simulink model "Synchronous_Buck_Converter_V2016B"  (R2016b)
settings: Solver=VariableStepAuto  StartTime=0.0  StopTime=0.006  RelTol=1e-3
libraries: fl_lib x13, elec_lib x7, nesl_utility x5
settings Model: Creator=whl14  LastModifiedBy=whl14

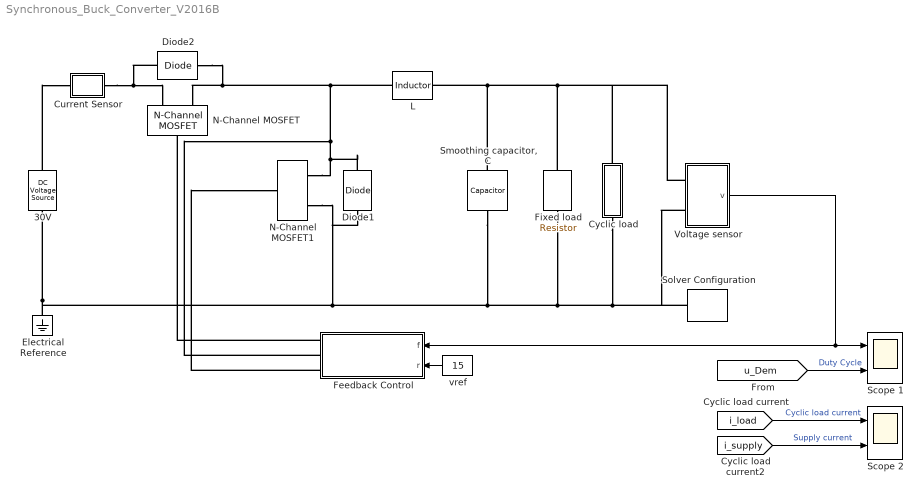
== system Synchronous_Buck_Converter_V2016B ==
  30V : fl_lib/Electrical/Electrical Sources/DC Voltage Source  v0=30 V
  Current Sensor : Subsystem
  Cyclic load : Subsystem
  Diode1 : elec_lib/Semiconductor Devices/Diode  ModelType=3  Vf=0.6 V  Ron=0.3 Ohm  Goff=1e-8 S  Rz=0.3 Ohm  Vz=50 V  C_PWL=5 pF  prmExp=1  I12=[ 0.25 5 ] A  V12=[ 0.7 0.8 ] V  I1=0.0137 A  V1=0.6 V  RS=0.01 Ohm  IS=1e-12 A  Tmeas=25 degC  ec=1  BV=Inf V  C_param=1  CJ0=5 pF  VJ=1 V  Mgrad=0.5  Vvec=[ 0.1 10 100 ] V  Cvec=[ 3.5 1 0.4 ] pF  FC=0.5  Q_param=1  Irrm=-7.15 A  iF=4 A  didt=-750 A/us  trr=115 ns  TT=50 ns  tau=100 ns  T_param=1  IS_T2=1.25e-7 A  I1_T2=0.245 A  V1_T2=0.5 V  Tmeas2=125 degC  EG_param=1  EG=1.11 eV  XTI_param=1  XTI=3  dBVdT=0 V/K  Tdevice=25 degC  Rth=[ 0 10 ] K/W  thermal_mass_parameterization=1  thermal_mass=[ 0 1 ] J/K  thermal_time_constant=[ 0 10 ] s  thermal_mass_initial_temperatures=[ 25 25 ] degC
  Diode2 : elec_lib/Semiconductor Devices/Diode  ModelType=3  Vf=0.6 V  Ron=0.3 Ohm  Goff=1e-8 S  Rz=0.3 Ohm  Vz=50 V  C_PWL=5 pF  prmExp=1  I12=[ 0.25 5 ] A  V12=[ 0.7 0.8 ] V  I1=0.0137 A  V1=0.6 V  RS=0.01 Ohm  IS=1e-12 A  Tmeas=25 degC  ec=1  BV=Inf V  C_param=1  CJ0=5 pF  VJ=1 V  Mgrad=0.5  Vvec=[ 0.1 10 100 ] V  Cvec=[ 3.5 1 0.4 ] pF  FC=0.5  Q_param=1  Irrm=-7.15 A  iF=4 A  didt=-750 A/us  trr=115 ns  TT=50 ns  tau=100 ns  T_param=1  IS_T2=1.25e-7 A  I1_T2=0.245 A  V1_T2=0.5 V  Tmeas2=125 degC  EG_param=1  EG=1.11 eV  XTI_param=1  XTI=3  dBVdT=0 V/K  Tdevice=25 degC  Rth=[ 0 10 ] K/W  thermal_mass_parameterization=1  thermal_mass=[ 0 1 ] J/K  thermal_time_constant=[ 0 10 ] s  thermal_mass_initial_temperatures=[ 25 25 ] degC
  Electrical Reference : fl_lib/Electrical/Electrical Elements/Electrical Reference
  Feedback Control : Subsystem  mask{Kp=0.5, Ki=200}
      mask init:
      | Kp=0.5
      | Ki=200
  Fixed load : fl_lib/Electrical/Electrical Elements/Resistor  R=3.75 Ohm  i_specify=off  i_priority=None  i=0 A  v_specify=off  v_priority=None  v=0 V
  L : fl_lib/Electrical/Electrical Elements/Inductor  l=1e-3 H  r=0 Ohm  g=0 1/Ohm  i_specify=off  i_priority=None  i=0 A  v_specify=off  v_priority=None  v=0 V  i_L_specify=off  i_L_priority=High  i_L=0 A
      settings: LogSimulationData=on
  N-Channel MOSFET : elec_lib/Semiconductor Devices/N-Channel MOSFET  parameterization=1  prmDatasheet=2  prmEquCoeff=1  Beta=5 A/V^2  Rds=0.1 Ohm  Id=6 A  Vgs=15 V  Vth=2 V  lam=0 1/V  Tmeas=25 degC  RS=0.01 Ohm  RD=0.01 Ohm  C_param=1  C_GS=270 pF  C_GD=80 pF  C_DS=0 pF  C_iss=350 pF  C_rss=80 pF  C_oss=0 pF  C_GS_vec=[ 270 300 290 280 295 255 ] pF  C_GD_vec=[ 450 400 300 190 95 55 ] pF  C_DS_vec=[ 450 410 390 230 175 115 ] pF  C_iss_vec=[ 720 700 590 470 390 310 ] pF  C_rss_vec=[ 450 400 300 190 95 55 ] pF  C_oss_vec=[ 900 810 690 420 270 170 ] pF  C_Vds_vec=[ 0.1 0.3 1 3 10 30 ] V  charge_linearity_param=1  C_OX=200 pF  V_C_OX=-0.5 V  IsDiode=0 A  Vbi=0.6 V  n=1  Cj0Diode=0 pF  TT=50e-9 s  dVth_dT=-6 mV/K  Rds_T2=0.2 Ohm  Tmeas2=125 degC  BEXDatasheet=-1.5  BEXEquCoeff=-1.5  etaisDatasheet=3  etaisEquCoeff=3  TdeviceDatasheet=T_junction1 degC  TdeviceEquCoeff=25 degC  Rth=[1.0, 10.0] K/W  thermal_mass_parameterization=1  thermal_mass=[1.0, 1.0] J/K  thermal_time_constant=[1.0, 10.0] s  thermal_mass_initial_temperatures=[ 25 25 ] degC  betaref=18 A/V^2  Vfbref=-1.1 V  gamma=3.5 V^0.50000  phib2ref=1 V  thesatref=0.4 1/V  alpha=0  Vp=5e-2 V  m=8  Tref=25 degC  Cox=1500 pF  Cgso=100 pF  Cgdo=14 pF  Rsref=2e-3 Ohm  Rdref=0.17 Ohm  Rgref=8.4 Ohm  Isref=5.2e-13 A  Cj0=480 pF  Tprm=1  etabet=1.3  Stvfb=5e-4 V/K  Stphib=-8.5e-4 V/K  etasat=1.04  etar=0.95  etais=3  Tsim=25 degC  T0=[25.0, 25.0] degC
  N-Channel MOSFET1 : elec_lib/Semiconductor Devices/N-Channel MOSFET  parameterization=1  prmDatasheet=1  prmEquCoeff=1  Beta=5 A/V^2  Rds=0.1 Ohm  Id=6 A  Vgs=15 V  Vth=2 V  lam=0 1/V  Tmeas=25 degC  RS=1e-4 Ohm  RD=0.01 Ohm  C_param=1  C_GS=270 pF  C_GD=80 pF  C_DS=0 pF  C_iss=350 pF  C_rss=80 pF  C_oss=0 pF  C_GS_vec=[ 270 300 290 280 295 255 ] pF  C_GD_vec=[ 450 400 300 190 95 55 ] pF  C_DS_vec=[ 450 410 390 230 175 115 ] pF  C_iss_vec=[ 720 700 590 470 390 310 ] pF  C_rss_vec=[ 450 400 300 190 95 55 ] pF  C_oss_vec=[ 900 810 690 420 270 170 ] pF  C_Vds_vec=[ 0.1 0.3 1 3 10 30 ] V  charge_linearity_param=1  C_OX=200 pF  V_C_OX=-0.5 V  IsDiode=0 A  Vbi=0.6 V  n=1  Cj0Diode=0 pF  TT=50e-9 s  dVth_dT=-6 mV/K  Rds_T2=0.037 Ohm  Tmeas2=125 degC  BEXDatasheet=-1.5  BEXEquCoeff=-1.5  etaisDatasheet=3  etaisEquCoeff=3  TdeviceDatasheet=25 degC  TdeviceEquCoeff=25 degC  Rth=[1.0, 10.0] K/W  thermal_mass_parameterization=1  thermal_mass=[1.0, 1.0] J/K  thermal_time_constant=[1.0, 10.0] s  thermal_mass_initial_temperatures=[ 25 25 ] degC  betaref=18 A/V^2  Vfbref=-1.1 V  gamma=3.5 V^0.50000  phib2ref=1 V  thesatref=0.4 1/V  alpha=0  Vp=5e-2 V  m=8  Tref=25 degC  Cox=1500 pF  Cgso=100 pF  Cgdo=14 pF  Rsref=2e-3 Ohm  Rdref=0.17 Ohm  Rgref=8.4 Ohm  Isref=5.2e-13 A  Cj0=480 pF  Tprm=1  etabet=1.3  Stvfb=5e-4 V/K  Stphib=-8.5e-4 V/K  etasat=1.04  etar=0.95  etais=3  Tsim=25 degC  T0=[25.0, 25.0] degC
  Scope 1 : Scope  NumInputPorts=2
  Scope 2 : Scope  NumInputPorts=2
  "Smoothing capacitor, C" : fl_lib/Electrical/Electrical Elements/Capacitor  c=22 uF  r=0 Ohm  g=0 1/Ohm  i_specify=off  i_priority=None  i=0 A  v_specify=off  v_priority=None  v=0 V  vc_specify=on  vc_priority=High  vc=0 V
  Solver Configuration : nesl_utility/Solver Configuration  PhysicalDomain=network_engine_domain  SubClassName=solver  LeftPortType=input  RightPortType=generic  Accelerate=off  Tones=[]  Harmonics=[]  SimulateNoise=off  Profile=off  UseLocalSampling=off  EnableSwitchedLinearOptims=on  FrequencyDomain=off  UseCCode=off  RelTol=0.001  AbsTol=1e-06  MinStep=1e-09  ToWorkspace=off  RevertToSquareIcSolve=off  NumHomotopyIterations=100  PhasorMode=off  PhasorModeNumHarmonics=1  OverrideAbsTol=off  DoDC=off  ResidualTolerance=1e-09  UseLocalSolver=off  LocalSolverChoice=NE_BACKWARD_EULER_ADVANCER  LocalSolverSampleTime=0.001  DoFixedCost=off  MaxNonlinIter=3  MaxModeIter=2  LinearAlgebra=Sparse  DelaysMemoryBudget=1024  AutomaticFiltering=on  FilteringTimeConstant=0.001
  Voltage sensor : Subsystem
  vref : Constant  Value=15
  wires:
  Voltage sensor/1(v) -> Feedback Control/1(f), Scope 1/1
  [i_load] -> Scope 2/1  "Cyclic load current"
  [i_supply] -> Scope 2/2  "Supply current"
  [u_Dem] -> Scope 1/2  "Duty Cycle"
  vref/1 -> Feedback Control/2(r)
  connections:
  Current Sensor/RConn1 -- Diode2/RConn1 -- N-Channel MOSFET/RConn1
  30V/LConn1 -- Current Sensor/LConn1
  N-Channel MOSFET1/RConn1 -- Diode1/RConn1 -- Feedback Control/RConn2 -- L/LConn1 -- Diode2/LConn1 -- N-Channel MOSFET/RConn2
  Electrical Reference/LConn1 -- "Smoothing capacitor, C"/RConn1 -- Fixed load/RConn1 -- Voltage sensor/LConn2 -- Solver Configuration/RConn1 -- Cyclic load/LConn1 -- Diode1/LConn1 -- N-Channel MOSFET1/RConn2 -- 30V/RConn1
  "Smoothing capacitor, C"/LConn1 -- Voltage sensor/LConn1 -- Cyclic load/RConn1 -- Fixed load/LConn1 -- L/RConn1
  Feedback Control/RConn1 -- N-Channel MOSFET/LConn1
  Feedback Control/RConn3 -- N-Channel MOSFET1/LConn1

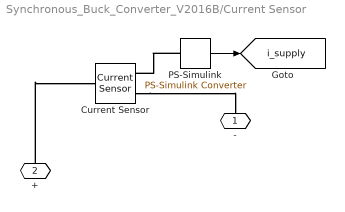
== system Synchronous_Buck_Converter_V2016B/Current Sensor ==
  Current Sensor : fl_lib/Electrical/Electrical Sensors/Current Sensor
  PS-Simulink : nesl_utility/PS-Simulink Converter  PhysicalDomain=network_engine_domain  SubClassName=ps_output  LeftPortType=input  RightPortType=output  PseudoPeriodic=off  Frequencies=[]  Unit=1  AffineConversion=off
  - : PMIOPort  Port=1  Side=Right
  + : PMIOPort  Port=2  Side=Left
  tag scope: i_supply=global
  wires:
  PS-Simulink/1 -> [i_supply]
  connections:
  Current Sensor/RConn2 -- -/RConn1
  PS-Simulink/LConn1 -- Current Sensor/RConn1
  +/RConn1 -- Current Sensor/LConn1

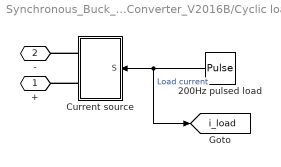
== system Synchronous_Buck_Converter_V2016B/Cyclic load ==
  200Hz pulsed load : DiscretePulseGenerator  PulseType=Time based  Period=1/200  PulseWidth=50  PhaseDelay=1/400
  Current source : Subsystem
  "+ " : PMIOPort  Port=1  Side=Right
  - : PMIOPort  Port=2  Side=Left
  tag scope: i_load=global
  wires:
  200Hz pulsed load/1 -> [i_load], Current source/1(S)  "Load current"
  connections:
  Current source/RConn2 -- "+ "/RConn1
  Current source/RConn1 -- -/RConn1

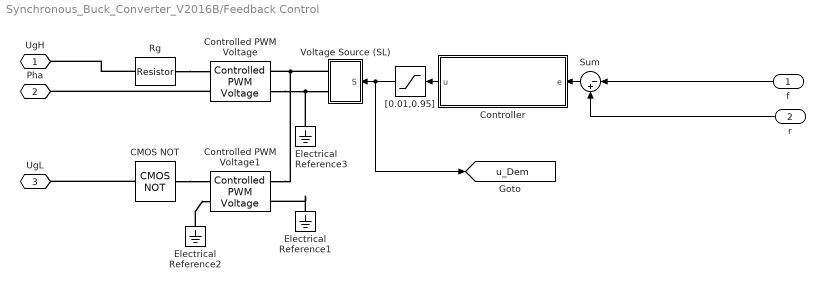
== system Synchronous_Buck_Converter_V2016B/Feedback Control ==
  f : Inport
  r : Inport  Port=2
  CMOS NOT : elec_lib/Integrated Circuits/Logic/CMOS NOT  V_IL=2 V  V_IH=3 V  C_IN=5 pF  output_type=1  V_OL=0 V  V_OH=5 V  V_CC=5 V  V_meas=5 V  R_OUT=25 Ohm  R_OH=[ 25 250 ] Ohm  I_OH=63 mA  R_OL=[ 30 800 ] Ohm  I_OL=-45 mA  Delay=25 ns  Ron=5 Ohm  Vf=0.6 V  output_state=1
  Controlled PWM Voltage : elec_lib/Actuators & Drivers/Drivers/Controlled PWM Voltage  F=50 kHz  TD=0 s  pulse_width_offset=0 s  Vmin=0 V  Vmax=1 V  Vm=30 V  pwm_or_av=1  event_type=1  sample_time=1e-6 s
  Controlled PWM Voltage1 : elec_lib/Actuators & Drivers/Drivers/Controlled PWM Voltage  F=50 kHz  TD=0 s  pulse_width_offset=0 s  Vmin=0 V  Vmax=1 V  Vm=30 V  pwm_or_av=1  event_type=1  sample_time=1e-6 s
  Controller : Subsystem  Variant=on  OverrideUsingVariant=controller_choice==1
      settings: AttributesFormatString=%<BlockChoice>
  Electrical Reference1 : fl_lib/Electrical/Electrical Elements/Electrical Reference
  Electrical Reference2 : fl_lib/Electrical/Electrical Elements/Electrical Reference
  Electrical Reference3 : fl_lib/Electrical/Electrical Elements/Electrical Reference
  Rg : fl_lib/Electrical/Electrical Elements/Resistor  R=100 Ohm  i_specify=off  i_priority=None  i=0 A  v_specify=off  v_priority=None  v=0 V
  Sum : Sum  Inputs=|-+
  Voltage Source (SL) : Subsystem
      settings: CopyFcn=set_param(gcb,'LinkStatus','none')
  "[0.01,0.95]" : Saturate  UpperLimit=0.95  LowerLimit=.01
  UgH : PMIOPort  Port=1  Side=Right
  Pha : PMIOPort  Port=2  Side=Right
  UgL : PMIOPort  Port=3  Side=Right
  tag scope: u_Dem=global
  wires:
  f/1 -> Sum/1
  Controller/1(u) -> "[0.01,0.95]"/1
  Sum/1 -> Controller/1(e)
  r/1 -> Sum/2
  "[0.01,0.95]"/1 -> [u_Dem], Voltage Source (SL)/1(S)
  connections:
  Controlled PWM Voltage/RConn2 -- Pha/RConn1
  Electrical Reference2/LConn1 -- Controlled PWM Voltage1/RConn2
  Voltage Source (SL)/RConn1 -- Controlled PWM Voltage1/LConn1 -- Controlled PWM Voltage/LConn1
  Rg/LConn1 -- Controlled PWM Voltage/RConn1
  Electrical Reference1/LConn1 -- Controlled PWM Voltage1/LConn2
  Rg/RConn1 -- UgH/RConn1
  CMOS NOT/LConn1 -- Controlled PWM Voltage1/RConn1
  Controlled PWM Voltage/LConn2 -- Electrical Reference3/LConn1 -- Voltage Source (SL)/RConn2
  CMOS NOT/RConn1 -- UgL/RConn1

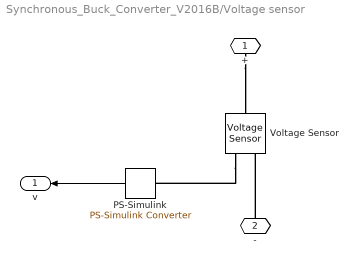
== system Synchronous_Buck_Converter_V2016B/Voltage sensor ==
  PS-Simulink : nesl_utility/PS-Simulink Converter  PhysicalDomain=network_engine_domain  SubClassName=ps_output  LeftPortType=input  RightPortType=output  PseudoPeriodic=off  Frequencies=[]  Unit=V  AffineConversion=off
  Voltage Sensor : fl_lib/Electrical/Electrical Sensors/Voltage Sensor
  + : PMIOPort  Port=1  Side=Left
  - : PMIOPort  Port=2  Side=Left
  v : Outport
  wires:
  PS-Simulink/1 -> v/1
  connections:
  +/RConn1 -- Voltage Sensor/LConn1
  -/RConn1 -- Voltage Sensor/RConn2
  Voltage Sensor/RConn1 -- PS-Simulink/LConn1

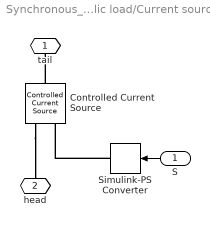
== system Synchronous_Buck_Converter_V2016B/Cyclic load/Current source ==
  S : Inport
  Controlled Current Source : fl_lib/Electrical/Electrical Sources/Controlled Current Source
  Simulink-PS Converter : nesl_utility/Simulink-PS Converter  PhysicalDomain=network_engine_domain  SubClassName=ps_input  LeftPortType=input  RightPortType=output  PseudoPeriodic=off  Frequencies=[]  NoiseDistribution=none  NoiseParameters=[]  Unit=1  AffineConversion=off  InputFiltering=off  SimscapeFilterOrder=1  InputFilterTimeConstant=0.001  UdotUserProvided=1
  tail : PMIOPort  Port=1  Side=Right
  head : PMIOPort  Port=2  Side=Right
  wires:
  S/1 -> Simulink-PS Converter/1
  connections:
  Simulink-PS Converter/RConn1 -- Controlled Current Source/RConn1
  Controlled Current Source/LConn1 -- tail/RConn1
  Controlled Current Source/RConn2 -- head/RConn1

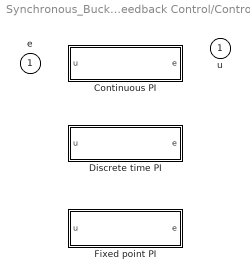
== system Synchronous_Buck_Converter_V2016B/Feedback Control/Controller ==
  e : Inport
  Continuous PI : Subsystem  VariantControl=controller_choice==1
  Discrete time PI : Subsystem  VariantControl=controller_choice==2
  Fixed point PI : Subsystem  MinMaxOverflowLogging=MinMaxAndOverflow  VariantControl=controller_choice==3
  u : Outport

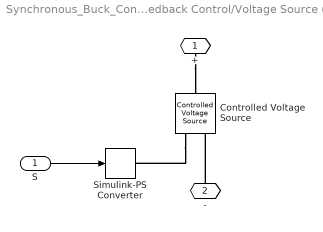
== system Synchronous_Buck_Converter_V2016B/Feedback Control/Voltage Source (SL) ==
  S : Inport
  Controlled Voltage Source : fl_lib/Electrical/Electrical Sources/Controlled Voltage Source
  Simulink-PS Converter : nesl_utility/Simulink-PS Converter  PhysicalDomain=network_engine_domain  SubClassName=ps_input  LeftPortType=input  RightPortType=output  PseudoPeriodic=off  Frequencies=[]  NoiseDistribution=none  NoiseParameters=[]  Unit=V  AffineConversion=off  InputFiltering=off  SimscapeFilterOrder=1  InputFilterTimeConstant=.001  UdotUserProvided=0
  + : PMIOPort  Port=1  Side=Right
  - : PMIOPort  Port=2  Side=Right
  wires:
  S/1 -> Simulink-PS Converter/1
  connections:
  +/RConn1 -- Controlled Voltage Source/LConn1
  -/RConn1 -- Controlled Voltage Source/RConn2
  Controlled Voltage Source/RConn1 -- Simulink-PS Converter/RConn1

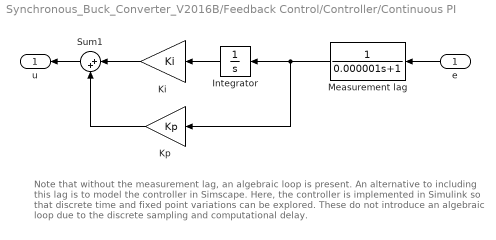
== system Synchronous_Buck_Converter_V2016B/Feedback Control/Controller/Continuous PI ==
  note: Note that without the measurement lag, an algebraic loop is present. An alternative to
      | including this lag is to model the controller in Simscape. Here, the controller is implemented
      | in Simulink so that discrete time and fixed point variations can be explored. These do not
      | introduce an algebraic loop due to the discrete sampling and computational delay.
  e : Inport
  Integrator : Integrator
  Ki : Gain  Gain=Ki
  Kp : Gain  Gain=Kp
  Measurement lag : TransferFcn  Denominator=[0.000001 1]
  Sum1 : Sum  Inputs=|++  SaturateOnIntegerOverflow=on  InputSameDT=on  OutDataTypeStr=Inherit: Same as first input
  u : Outport
  wires:
  Measurement lag/1 -> Integrator/1, Kp/1
  Ki/1 -> Sum1/1
  Sum1/1 -> u/1
  Kp/1 -> Sum1/2
  Integrator/1 -> Ki/1
  e/1 -> Measurement lag/1

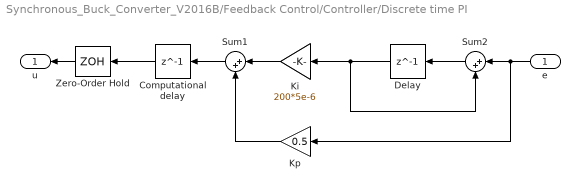
== system Synchronous_Buck_Converter_V2016B/Feedback Control/Controller/Discrete time PI ==
  e : Inport
  Computational delay : Delay  DelayLength=1  InputProcessing=Inherited  SampleTime=5e-6
  Delay : Delay  DelayLength=1  InputProcessing=Inherited  SampleTime=5e-6
  Ki : Gain  Gain=200*5e-6
  Kp : Gain  Gain=0.5
  Sum1 : Sum  Inputs=|++  SaturateOnIntegerOverflow=on  InputSameDT=on  OutDataTypeStr=Inherit: Same as first input
  Sum2 : Sum  Inputs=|++  SaturateOnIntegerOverflow=on  InputSameDT=on  OutDataTypeStr=Inherit: Same as first input
  Zero-Order Hold : ZeroOrderHold  SampleTime=5e-6
  u : Outport
  wires:
  Ki/1 -> Sum1/1
  Sum2/1 -> Delay/1
  Delay/1 -> Ki/1, Sum2/2
  Kp/1 -> Sum1/2
  Sum1/1 -> Computational delay/1
  e/1 -> Sum2/1, Kp/1
  Zero-Order Hold/1 -> u/1
  Computational delay/1 -> Zero-Order Hold/1

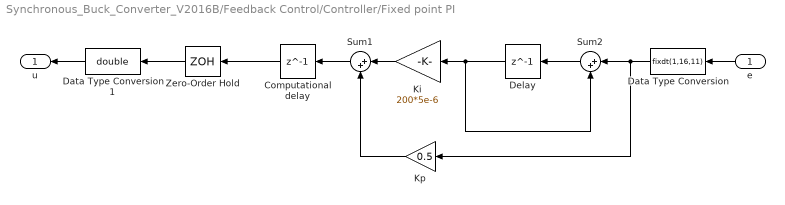
== system Synchronous_Buck_Converter_V2016B/Feedback Control/Controller/Fixed point PI ==
  e : Inport
  Computational delay : Delay  DelayLength=1  InputProcessing=Inherited  SampleTime=5e-6
  Data Type Conversion : DataTypeConversion  OutDataTypeStr=fixdt(1,16,11)  RndMeth=Nearest
  Data Type Conversion1 : DataTypeConversion  OutDataTypeStr=double  RndMeth=Nearest
  Delay : Delay  DelayLength=1  InputProcessing=Inherited  SampleTime=5e-6
  Ki : Gain  Gain=200*5e-6  OutDataTypeStr=fixdt(1,16,13)  RndMeth=Nearest
  Kp : Gain  Gain=0.5  OutDataTypeStr=fixdt(1,16,9)  RndMeth=Nearest
  Sum1 : Sum  Inputs=|++  SaturateOnIntegerOverflow=on
  Sum2 : Sum  Inputs=|++  SaturateOnIntegerOverflow=on  InputSameDT=on  OutDataTypeStr=Inherit: Same as first input
  Zero-Order Hold : ZeroOrderHold  SampleTime=5e-6
  u : Outport
  wires:
  Ki/1 -> Sum1/1
  Data Type Conversion1/1 -> u/1
  Data Type Conversion/1 -> Sum2/1, Kp/1
  Sum1/1 -> Computational delay/1
  Kp/1 -> Sum1/2
  e/1 -> Data Type Conversion/1
  Delay/1 -> Ki/1, Sum2/2
  Sum2/1 -> Delay/1
  Computational delay/1 -> Zero-Order Hold/1
  Zero-Order Hold/1 -> Data Type Conversion1/1
